simulink model "tilt_system"  (Simulink 8.5)
settings: Solver=FixedStepDiscrete  StartTime=0.0  StopTime=10  FixedStep=0.01  RelTol=1e-3
PreLoadFcn:
  | seed1 = 1
  | seed2 = 2
libraries: simulink x4
settings Model: Creator=Administrator  LastModifiedBy=James
settings DebuggingCC: SolverPrmCheckMsg=warning  FcnCallInpInsideContextMsg=UseLocalSettings  StrictBusMsg=Warning

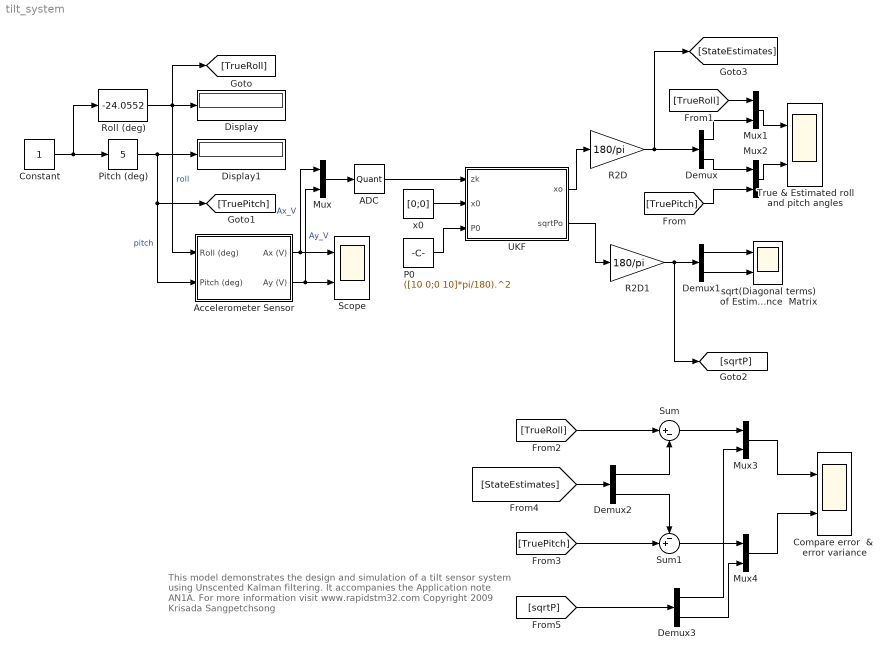
== system tilt_system ==
  note: This model demonstrates the design and simulation
      | of a tilt sensor system using Unscented Kalman filtering.
      | It accompanies the Application note AN1A.
      | For more information visit www.rapidstm32.com
      |
      | Copyright 2009 Krisada Sangpetchsong
  ADC : Quantizer  QuantizationInterval=3.3/2^12
  Accelerometer Sensor : Subsystem
  Compare error  &  error variance : Scope  NumInputPorts=2
      settings: TimeRange=10  YMin=-0.8~-0.15  YMax=0.2~0.2  SaveName=error_variance
  Constant : Constant
  Demux{,1..3} (4 alike) : Demux  Outputs=2
  Display : Display
  Display1 : Display
  Mux{,1..4} (5 alike) : Mux  Inputs=2
  P0 : Constant  Value=([10 0;0 10]*pi/180).^2
  Pitch (deg) : simulink/Math Operations/Slider Gain  low=-90  gain=5  high=90
  R2D : Gain  Gain=180/pi
  R2D1 : Gain  Gain=180/pi
  Roll (deg) : simulink/Math Operations/Slider Gain  low=-180  gain=-24.0552  high=180
  Scope : Scope  NumInputPorts=2
      settings: YMin=-0.0015~-0.075  YMax=0.0015~0.2
  Sum : Sum  Inputs=|+-
  Sum1 : Sum  Inputs=-+|
  True & Estimated roll and pitch angles : Scope  NumInputPorts=2
      settings: YMin=-24.2~-0.5  YMax=-23.7~5.5
  UKF : MATLAB Function  TreatAsAtomicUnit=on
  sqrt(Diagonal terms) of Estimation  Error Covariance  Matrix : Scope  NumInputPorts=2
      settings: YMin=-5~-5  YMax=5~5  SaveName=ScopeData2
  x0 : Constant  Value=[0;0]
  wires:
  Constant/1 -> Roll (deg)/1, Pitch (deg)/1
  Roll (deg)/1 -> Display/1, [TrueRoll], Accelerometer Sensor/1(Roll (deg))  "roll"
  Pitch (deg)/1 -> Display1/1, [TruePitch], Accelerometer Sensor/2(Pitch (deg))  "pitch"
  Mux/1 -> ADC/1
  ADC/1 -> UKF/1(zk)
  x0/1 -> UKF/2(x0)
  P0/1 -> UKF/3(P0)
  UKF/1(xo) -> R2D/1
  UKF/2(sqrtPo) -> R2D1/1
  R2D1/1 -> Demux1/1, [sqrtP]
  [TrueRoll] -> Mux1/1
  R2D/1 -> Demux/1, [StateEstimates]
  Demux/1 -> Mux1/2
  Demux/2 -> Mux2/1
  [TruePitch] -> Mux2/2
  Demux1/1 -> sqrt(Diagonal terms) of Estimation  Error Covariance  Matrix/1
  Demux1/2 -> sqrt(Diagonal terms) of Estimation  Error Covariance  Matrix/2
  Mux1/1 -> True & Estimated roll and pitch angles/1
  Mux2/1 -> True & Estimated roll and pitch angles/2
  Accelerometer Sensor/1(Ax (V)) -> Scope/1, Mux/1  "Ax_V"
  Accelerometer Sensor/2(Ay (V)) -> Scope/2, Mux/2  "Ay_V"
  [StateEstimates] -> Demux2/1
  [TruePitch] -> Sum1/2
  Demux2/2 -> Sum1/1
  Demux2/1 -> Sum/2
  [TrueRoll] -> Sum/1
  [sqrtP] -> Demux3/1
  Sum/1 -> Mux3/1
  Sum1/1 -> Mux4/1
  Demux3/1 -> Mux3/2
  Demux3/2 -> Mux4/2
  Mux3/1 -> Compare error  &  error variance/1
  Mux4/1 -> Compare error  &  error variance/2

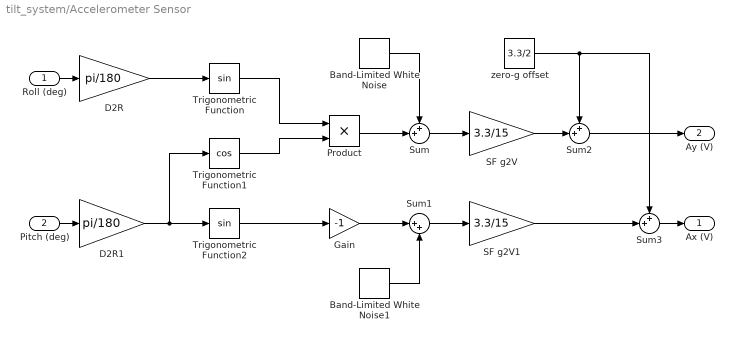
== system tilt_system/Accelerometer Sensor ==
  Roll (deg) : Inport
  Pitch (deg) : Inport  Port=2
  Band-Limited White Noise : simulink/Sources/Band-Limited White Noise  SystemSampleTime=-1  Cov=(.002^2)*0.01  Ts=0.01  seed=seed1
  Band-Limited White Noise1 : simulink/Sources/Band-Limited White Noise  SystemSampleTime=-1  Cov=(.002^2)*0.01  Ts=0.01  seed=seed2
  D2R : Gain  Gain=pi/180
  D2R1 : Gain  Gain=pi/180
  Gain : Gain  Gain=-1
  Product : Product  RndMeth=Zero
  SF g2V : Gain  Gain=3.3/15
  SF g2V1 : Gain  Gain=3.3/15
  Sum : Sum  Inputs=++|
  Sum1 : Sum  Inputs=|++
  Sum2 : Sum  Inputs=++|
  Sum3 : Sum  Inputs=++|
  Trigonometric Function : Trigonometry
  Trigonometric Function1 : Trigonometry  Operator=cos
  Trigonometric Function2 : Trigonometry
  zero-g offset : Constant  Value=3.3/2
  Ax (V) : Outport
  Ay (V) : Outport  Port=2
  wires:
  Band-Limited White Noise1/1 -> Sum1/2
  Product/1 -> Sum/2
  Gain/1 -> Sum1/1
  Band-Limited White Noise/1 -> Sum/1
  Trigonometric Function2/1 -> Gain/1
  Trigonometric Function/1 -> Product/1
  Trigonometric Function1/1 -> Product/2
  D2R1/1 -> Trigonometric Function1/1, Trigonometric Function2/1
  D2R/1 -> Trigonometric Function/1
  Sum1/1 -> SF g2V1/1
  Sum/1 -> SF g2V/1
  SF g2V/1 -> Sum2/2
  SF g2V1/1 -> Sum3/2
  zero-g offset/1 -> Sum3/1, Sum2/1
  Roll (deg)/1 -> D2R/1
  Sum2/1 -> Ay (V)/1
  Pitch (deg)/1 -> D2R1/1
  Sum3/1 -> Ax (V)/1

== matlab function UKF ==
  data: zk input double; xo output double; x0 input double; P0 input double; sqrtPo output double
% Unscented Kalman Filtering source code for Tilt Sensor System
% To be implemented in the  Embedded MATLAB Function block
%
% An example for Rapid STM32 Blockset 
%
% Application Note AN1 Developing a Tilt Sensor System Using Rapid STM32 Blockset
%
% Copyright 2009 Krisada Sangpetchsong
%
% Visit  www.rapidstm32.com for further information
  
function [xo, sqrtPo] = tilt_sensor_ukf(zk, x0, P0)
 
% Input
% zk   Measurements zk = [Ax; Ay] in volts
% x0   Initial state estimate 
% P0   Initial error covariance matrix
%
% Output
% xo   State estimate xo = [roll; pitch] in radians
% sqrtPo  Square root of the diagonal term of the estimation error covariance matrix
 
persistent x % State vector x = [roll; pitch]
persistent P % Error covariance matrix
persistent Qk % Driving noise covariance matrix
persistent Rk % Measurement noise covariance matrix
persistent Xm % Temporary buffer for predicted state sigma points
persistent Z % Temporary buffer for predicted measurement sigma points
 
% Initialise persistent parameters
% persistent variable in m-file is the same as static variable in C
if isempty(x)
    x = x0;
end
if isempty(P)
    P = P0;
end
if isempty(Qk)
    Qk = [1e-7 0; 0 1e-7];  % must be modified to match your model.
    % in rad^2 choosen arbitrary to prevent divergence 
    % due to numerical instability
end
if isempty(Rk)
    Rk = [2e-3 0; 0 2e-3].^2;  % must be modified to match your model.
    % in g^2
end
if isempty(Xm)
    Xm = zeros(2,4);    % must be modified to match your model.
    % Xm = zeros(nbr_row,nbr_col); 
    % nbr_row = number of row of the state vector x i.e. n
    % when x = [roll; pitch], n = 2
    % nbr_col = n * 2 = 2 * 2 = 4 
end
if isempty(Z)
    Z = zeros(2,4);  % must be modified to match your model.
    % Z = zeros(nbr_row,nbr_col); 
    % nbr_row = number of measurements i.e. when zk = [Ax, Ay], nbr_row = 2
    % nbr_col = n * 2 i.e. when x = [roll; pitch], nbr_col = 2*2 = 4
end
 
% Umrechnung nicht bei jedem System
% Convert measurements from volts to g
% must be modified to match your model.
SF = 15/3.3; % Scale factor is 15/Vdd g/V for LIS3L06AQ +/-6g full scale 
A0 = 3.3/2; % Zero-g offset Vdd/2
zk_g = SF*(zk-A0);

% Start UKF Routine
%---------------------------------------------------------------
% Find sigma points X
X = ukf_sigmapoints(x,P);
n2 = size(X,2); % Size of the state vector multiplied by 2
 
% Predicted states for next time step computed from the sigma points X
for k = 1:n2
    Xm(:,k) = updatex(X(:,k)); % Wenn updatex_RungeKutta vewendet wird in Zeile 131 dann muss der Ausdruck updatex angepasst werden.
end
 
% Find the prediction mean and covariance matrix
[xm, Pm] = ukf_mean_covariance(Xm);
Pm = Pm + Qk;
 
% Predicted measurements sigma points
for k = 1:n2
    Z(:,k) = h(Xm(:,k)); % must be modified to match your model (only if the h function has more input or output parameters).
end
 
% Find mean and covariance
[z, Pz] = ukf_mean_covariance(Z);
Pz = Pz + Rk;
 
Pxz = ukf_covariance(Xm, Z); % Cross covariance matrix
 
Kk = Pxz/Pz; % Kalman gain matrix
x = xm + Kk*(zk_g - z); % Find the state estimates
P = Pm - Kk*Pz*Kk'; % Estimation error covariance matrix
P = 0.5*(P+P'); % Prevent numerical problem
 
xo = x;
sqrtPo = sqrt(diag(P));
 
% end tilt_sensor_ukf
 
%--------------------------------------------------
% This is the nonlinear measurement model
% This function h(x) must be modified to match your measurement model.
function z = h(x)
 
z1 = -sin(x(2));
z2 = sin(x(1))*cos(x(2));
z = [z1; z2];
 
%--------------------------------------------------
% This function is used to propagate the state vector 
% from time step tk to tk+1.
% In our tilt sensor system the propagation is quite simple
% since we are estimating constants.
% This function updatex (x) must be modified to match your process model.
function xo = updatex(x)
 
% From F = [0 0; 0 0]
% expm(F) = [1 0; 0 1];
% i.e. xo(1) = x(1), xo(2) = x(2), ...
xo = x;
 
% If the process model is highly nonlinear, 
% it is possible to use more accurate numerical integration techniques
% such as 4th order Runge Kutta method to propagate the states.
%
% Example: 4th order Runge Kutta Update Routine
% function xo = updatex_RungeKutta(x, dt, varin)
% 
% varin is the input arguments
% dt is the sample time (tk+1 - tk)
%
% h_by2 = 0.5*dt;
% k1 = fx(x, varin);
% k2 = fx(x + k1*h_by2, varin);
% k3 = fx(x + k2*h_by2, varin);
% k4 = fx(x + k3*h_by2, varin);
% xo = x + (h/6)*(k1 +2*(k2 + k3) + k4);
%
% where the nonlinear differential equations are defined as follows.
%
% function dx = fx(x, varin)
% 
% dx1 = f1(x,varin);
% dx2 = f2(x,varin);
% ...
% dx = [dx1; dx2; ...]
 
%%%%%%%%%%%%%%%%%%%%%%%%%%%%%%%%%%%%%%%%%%%%%%%%%%%
% It is not necessary to modify the following three functions AT ALL.
% function X = ukf_sigmapoints(xbar,Pi)
% function [m, P] = ukf_mean_covariance(sigmaX)
% function P = ukf_covariance(sigmaX, sigmaY)
% These functions can be used in any UKF systems.
%%%%%%%%%%%%%%%%%%%%%%%%%%%%%%%%%%%%%%%%%%%%%%%%%%%
%--------------------------------------------------
% This function is used to compute the sigma points
% Input 
% xbar   is the mean value of x
% Pi     is the associated covariance matrix
%
% Output
% X is the sigma points
% The size of X is determined as follows.
% The number of rows is the same as the number of rows of xbar i.e. n
% The number of columns is 2*n
% Optimal state estimation, Dan Simon, p. 446 ISBN 100471708585
function X = ukf_sigmapoints(xbar,Pi)
 
n = size(xbar,1);
A = chol(n*Pi)'; % R = chol(A) where R'*R = A
X = [A -A] + repmat(xbar,1,n*2);
 
%--------------------------------------------------
% This function computes the mean and covariance matrix from the sigma points.
% m is the mean computed from the sigma points.
% P is the covariance matrix computed from the sigma points and the mean.
function [m, P] = ukf_mean_covariance(sigmaX)
 
n2 = size(sigmaX,2);
m = sum(sigmaX,2)/n2;
P = zeros(size(sigmaX,1)); % size n
for k = 1:n2
    P = P + ((sigmaX(:,k)-m)*(sigmaX(:,k)-m)');
end
P = P/n2;
 
%--------------------------------------------------
% This function computes the cross covariance matrix from two sets of sigma points.
% P is the cross covariance matrix computed from the sigma points and the mean.
% sigmaX and sigmaY are the sigma points of X and Y respectively.
function P = ukf_covariance(sigmaX, sigmaY)
 
n2 = size(sigmaX,2); % 2*n
mx = sum(sigmaX,2)/n2;
my = sum(sigmaY,2)/n2;
P = zeros(size(sigmaX,1),size(sigmaY,1)); % size n
for k = 1:n2
    P = P + ((sigmaX(:,k)-mx)*(sigmaY(:,k)-my)');
end
P = P/n2;
